simulink model "Milestone_2_Simulation"  (R2021a)
settings: Solver=FixedStepDiscrete  StartTime=0.0  StopTime=4  FixedStep=0.01  RelTol=1e-3
values from neighbouring files (symbols this model uses):
  ticksPerRot =     [robotParameters.m]
  wheelR =     [robotParameters.m]
undefined symbols (not defined in the file or in its folder): InputPWM, WheelSpeed
libraries: mobileRoboticsTrainingLib x6
settings Model: EnablePacing=on  PacingRate=3  Creator=Boitumelo  LastModifiedBy=brennannaidoo

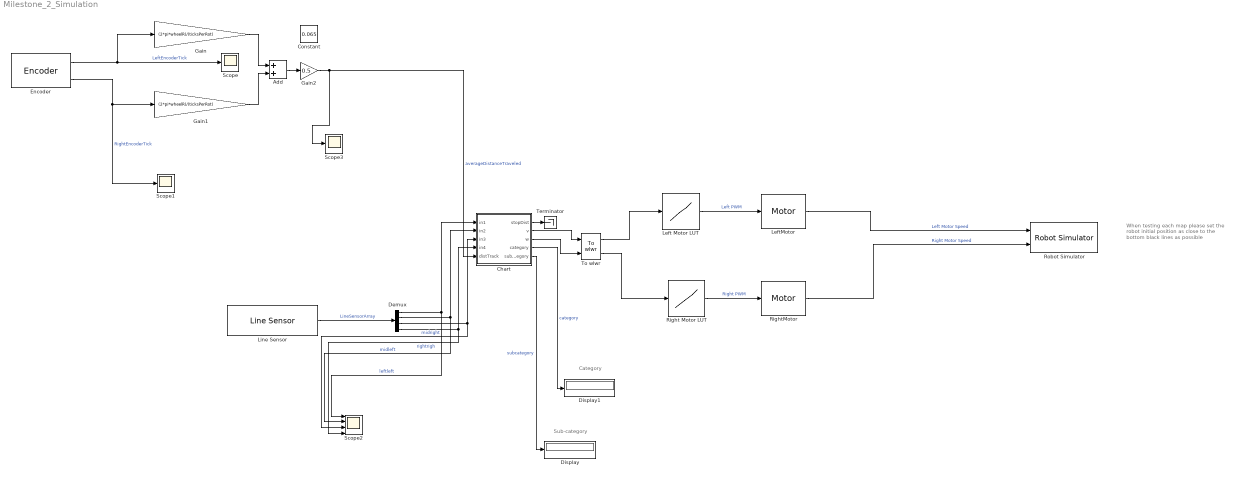
== system Milestone_2_Simulation ==
  note: When testing each map please
      | set the robot initial position as close
      | to the bottom black lines as possible
  note: Sub-category
  note: Category
  Add : Sum
  Chart : Stateflow chart  TreatAsAtomicUnit=on
  Constant : Constant  Value=0.065
  Demux : Demux
  Display : Display
  Display1 : Display
  Encoder : mobileRoboticsTrainingLib/Encoder  axleLength=axleLength  wheelR=wheelR  ticksPerRot=ticksPerRot
      settings: SourceProductName=Mobile Robotics Training Library
  Gain : Gain  Gain=(2*pi*wheelR)/(ticksPerRot)
  Gain1 : Gain  Gain=(2*pi*wheelR)/(ticksPerRot)
  Gain2 : Gain  Gain=0.5
  Left Motor LUT : Lookup_n-D  NumberOfTableDimensions=1  BreakpointsForDimension1=WheelSpeed  Table=InputPWM  InterpMethod=Nearest  ExtrapMethod=Clip  InternalRulePriority=Speed  RndMeth=Simplest  InputSameDT=on
  LeftMotor : mobileRoboticsTrainingLib/Motor  motorPlant=wheelMotorModel  sensorType=Speed
      settings: SourceProductName=Mobile Robotics Training Library
  Line Sensor : mobileRoboticsTrainingLib/Line Sensor  mapVariable=mapForSim  envVal=1  lineVal=0  sensOff=[0.0643 0.0354; 0.0675 0.005; 0.0675 -0.005; 0.0643 -0.0354]
      settings: SourceProductName=Mobile Robotics Training Library
  Right Motor LUT : Lookup_n-D  NumberOfTableDimensions=1  BreakpointsForDimension1=WheelSpeed  Table=InputPWM  InterpMethod=Nearest  ExtrapMethod=Clip  InternalRulePriority=Speed  RndMeth=Simplest  InputSameDT=on
  RightMotor : mobileRoboticsTrainingLib/Motor  motorPlant=wheelMotorModel  sensorType=Speed
      settings: SourceProductName=Mobile Robotics Training Library
  Robot Simulator : mobileRoboticsTrainingLib/Robot Simulator  Priority=99  mapVar=mapForSim  startX=0.21087  startY=0.11341  startTheta=90  axleLength=axleLength  wheelR=wheelR
  Scope : Scope
  Scope1 : Scope
  Scope2 : Scope  NumInputPorts=4
  Scope3 : Scope
  Terminator : Terminator
  To wlwr : mobileRoboticsTrainingLib/To wlwr  axleLength=0.1  wheelR=0.05
  wires:
  LeftMotor/1 -> Robot Simulator/1  "Left Motor Speed"
  RightMotor/1 -> Robot Simulator/2  "Right Motor Speed"
  Right Motor LUT/1 -> RightMotor/1  "Right PWM"
  Left Motor LUT/1 -> LeftMotor/1  "Left PWM"
  Encoder/1 -> Gain/1, Scope/1  "LeftEncoderTick"
  Encoder/2 -> Gain1/1, Scope1/1  "RightEncoderTick"
  To wlwr/1 -> Left Motor LUT/1
  To wlwr/2 -> Right Motor LUT/1
  Line Sensor/1 -> Demux/1  "LineSensorArray"
  Add/1 -> Gain2/1
  Gain/1 -> Add/1
  Gain1/1 -> Add/2
  Gain2/1 -> Chart/5(distTrack), Scope3/1  "averageDistanceTraveled"
  Demux/1 -> Scope2/1, Chart/1(in1)  "leftleft"
  Demux/2 -> Chart/2(in2), Scope2/2  "midleft"
  Demux/3 -> Chart/3(in3), Scope2/3  "midright"
  Demux/4 -> Scope2/4, Chart/4(in4)  "rightrigh"
  Chart/3(w) -> To wlwr/2
  Chart/1(stopDist) -> Terminator/1
  Chart/5(subcategory) -> Display/1  "subcategory"
  Chart/4(category) -> Display1/1  "category"
  Chart/2(v) -> To wlwr/1

== stateflow chart Milestone_2_Simulation/Chart ==
  note: Note the different distTrack conditions,
      | these were needed for the Category 2 junctions.
      | Values were done by hand (i.e simulating until a
      | satisfactory result was achieved in this case these
      | were:
      | (Normal)T-junction and Crossing - stop in middle of junction
      | End of Maze - Stop in end
      | Other- no significant stopping point was considered
      | for other junctions, if this is needed changes can
      | be quickly implemented via the stateflow logic
      | /tansition conditions as was done for the category
      | 2 junctions.
      |
      | Some overshoot exists in all situations because of
      | the chosen solution, it doesn't work well but atleast
      | it works.
  state EndOfMaze
    entry:
    v=0;
    w=0;
    subcategory= 1;
  state CrossRoads
    entry:
    v=0;
    w=0;
    subcategory= 2;
  note: Category 2 Junctions:
      | Normal T Junction
      | Fourway Crossing
      | End of Maze
  state Junction1_0000_
    entry:
    v=0.1;
    w =0;
    stopDist=0.018
    startDist = distTrack
    category = 2
  state TJunc
    entry:
    v=0;
    w=0;
    subcategory= 3;
  state Initial
    entry:
    v=0;
    w=0;
    stopDist=0;
    category= 0;
  state MoveForward
    v=0.1;
    w=0;
    stopDist=2
    category = 1
  state StartDetect
    entry:
    stopDist=0
  state Junction2_1000_
    entry:
    v=0.1;
    w=0;
    stopDist=0.018
    category = 3
  state RightTurn
    entry:
    v=0;
    w=0;
    subcategory= 1;
  state RightTJunc
    entry:
    v=0;
    w=0;
    subcategory= 2;
  state Junction3_0001_
    entry:
    v=0.1;
    w=0;
    stopDist=0.018
    category = 4
  state LeftTurn
    entry:
    v=0;
    w=0;
    subcategory= 1;
  state LeftTJunc
    entry:
    v=0;
    w=0;
    subcategory= 2;
  state DeadEnd
    entry:
    v=0;
    w=0;
    category = 5
    subcategory= 1;
  Junction1_0000_ -> EndOfMaze [order 1] : [distTrack >= (startDist + 0.075) & in1==0 & in2==0 & in3==0 & in4==0 ]
  Junction1_0000_ -> CrossRoads [order 2] : [distTrack >= (startDist + 0.075) & in1==1 & in2==0 & in3==0 & in4==1 ]
  MoveForward -> Junction1_0000_ [order 1] : [in1==0 & in2==0 & in3==0 & in4==0 ]
  (default) -> Initial
  Junction1_0000_ -> TJunc [order 3] : [distTrack >= (startDist + 0.059) & in1==1 & in2==1 & in3==1 & in4==1 ]
  StartDetect -> MoveForward : [in2==0 & in3==0]
  Initial -> StartDetect
  MoveForward -> Junction2_1000_ [order 2] : [in1==1 & in2==0 & in3==0 & in4==0]
  MoveForward -> DeadEnd [order 4] : [in1==1 & in2==1 & in3==1 & in4==1]
  MoveForward -> Junction3_0001_ [order 3] : [in1==0 & in2==0 & in3==0 & in4==1]
  Junction2_1000_ -> RightTurn [order 1] : [in1==1 & in2==1 & in3==1 & in4==1 ]
  Junction2_1000_ -> RightTJunc [order 2] : [in1==1 & in2==0 & in3==0 & in4==1 ]
  Junction3_0001_ -> LeftTurn [order 1] : [in1==1 & in2==1 & in3==1 & in4==1]
  Junction3_0001_ -> LeftTJunc [order 2] : [in1==1 & in2==0 & in3==0 & in4==1 ]
  data: stopDist output; in1 input; in2 input; in3 input; in4 input; v output; w output; category output; subcategory output; distTrack input; startDist local
